simulink model "Finishonlyautomomous_v1"  (R2023b)
settings: Solver=FixedStepAuto  StartTime=0.0  StopTime=inf  RelTol=1e-3
libraries: vexarmcortexlib x6, vexcommonlib x2
settings Model: SimulationMode=external  ExtModeTrigDuration=25  Creator=nicoa  LastModifiedBy=ierdn
settings SolverCC: AlgebraicLoopSolver=TrustRegion
settings OptimizationCC: EnhancedBackFolding=on  PassReuseOutputArgsAs=Individual arguments  ZeroExternalMemoryAtStartup=off  ZeroInternalMemoryAtStartup=off  MaxStackSize=64  OptimizeBlockOrder=speed  DifferentSizesBufferReuse=on  OptimizationCustomize=off  EfficientTunableParamExpr=on
settings DebuggingCC: ParameterTunabilityLossMsg=error  UnconnectedInputMsg=warning  UnconnectedOutputMsg=warning  UnconnectedLineMsg=warning
settings HardwareCC: ProdBitPerPointer=32  ProdBitPerSizeT=32  ProdBitPerPtrDiffT=32  ProdLargestAtomicInteger=Long  ProdLargestAtomicFloat=Double  ProdWordSize=32  ProdHWDeviceType=ARM Compatible->ARM Cortex
settings ModelReferenceCC: EnableRefExpFcnMdlSchedulingChecks=on
settings SFSimCC: MATLABDynamicMemAlloc=off
settings RTWCC: Description=Embedded Coder  SystemTargetFile=ert.tlc  HardwareBoard=ARM Cortex-based VEX Microcontroller  TLCOptions="-aInlineSetEventsForThisBaseRateFcn=TLC_FALSE -aSuppressMultiTaskScheduler=TLC_FALSE  -aRateBasedStepFcn=0"  TemplateMakefile=ert_default_tmf  GenerateReport=on  Toolchain=GNU Tools for VEX ARM Cortex  IncludeHyperlinkInReport=on  LaunchReport=on  GenerateTraceInfo=on  GenerateTraceReport=on  GenerateTraceReportSl=on  GenerateTraceReportSf=on  GenerateTraceReportEml=on
settings CodeAppCC: ForceParamTrailComments=on  IgnoreCustomStorageClasses=off  OperatorAnnotations=on  SimulinkDataObjDesc=on  SFDataObjDesc=on  InsertBlockDesc=on
settings ERTTargetCC: ExtMode=on  ExtModeTransport=1  ExtModeMexFile=ext_serial_win32_comm  ExtModeMexArgs=1 3 115200

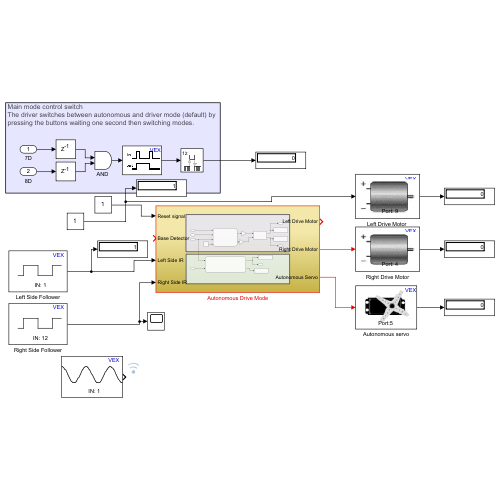
[thumbnail: Simulink's stored preview of the top-level diagram]
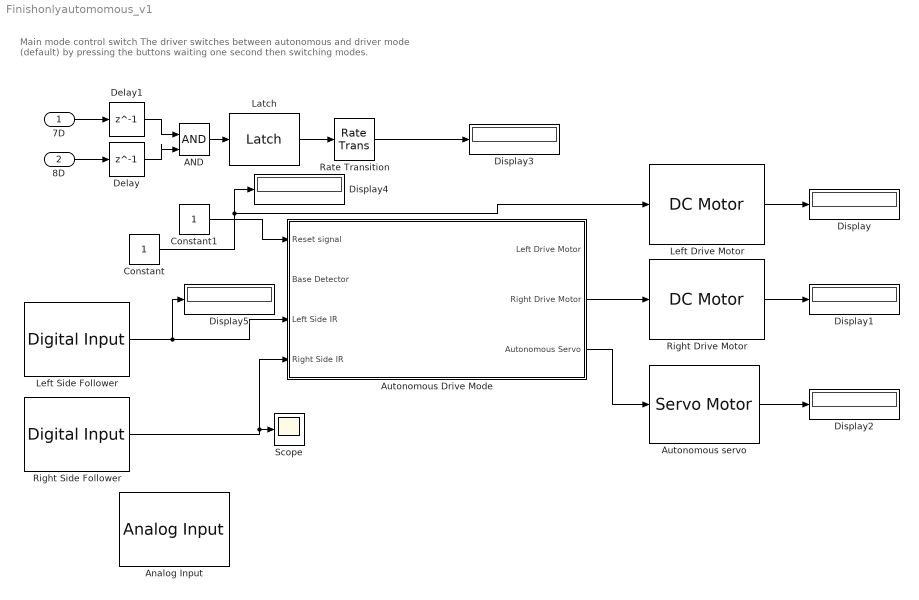
== system Finishonlyautomomous_v1 ==
  note: Main mode control switch
      | The driver switches between autonomous and driver mode (default) by
      | pressing the buttons waiting one second then switching modes.
  7D : Inport
  8D : Inport  Port=2
  "AND " : Logic  IconShape=distinctive  AllPortsSameDT=off  OutDataTypeStr=boolean
  Analog Input : vexarmcortexlib/Sensors/Analog Input  inChan=1  SimulationIn=off  SampleTime=0.05
  Autonomous Drive Mode : Subsystem
  Autonomous servo : vexarmcortexlib/Actuators/Servo Motor  motor=5  scaleFactor=60/127  SimulationOut=on
  Constant : Constant
  Constant1 : Constant
  Delay : Delay  DelayLength=1  InitialCondition=0  SampleTime=1
  Delay1 : Delay  DelayLength=1  InitialCondition=0  SampleTime=1
  Display{,1..5} (6 alike) : Display
  Latch : vexcommonlib/Latch  output0=off  BlockPlatform=vexarmcortex
  "Left Drive Motor " : vexarmcortexlib/Actuators/DC Motor  motor=9  scaleFactor=1/13.5  SimulationOut=on
  Left Side Follower : vexarmcortexlib/Sensors/Digital Input  inChan=1  SimulationIn=off  SampleTime=0.2
  Rate Transition : RateTransition
  Right Drive Motor : vexarmcortexlib/Actuators/DC Motor  motor=4  scaleFactor=1/13.5  SimulationOut=on
  Right Side Follower : vexarmcortexlib/Sensors/Digital Input  inChan=12  SimulationIn=off  SampleTime=0.2
  Scope : Scope
  wires:
  Delay1/1 -> "AND "/1
  "AND "/1 -> Latch/1
  7D/1 -> Delay1/1
  8D/1 -> Delay/1
  Latch/1 -> Rate Transition/1
  Delay/1 -> "AND "/2
  Right Side Follower/1 -> Scope/1, Autonomous Drive Mode/4(Right Side IR)
  Left Side Follower/1 -> Display5/1, Autonomous Drive Mode/3(Left Side IR)
  Constant/1 -> "Left Drive Motor "/1, Display4/1
  Autonomous Drive Mode/2(Right Drive Motor) -> Right Drive Motor/1
  Autonomous Drive Mode/3(Autonomous Servo) -> Autonomous servo/1
  "Left Drive Motor "/1 -> Display/1
  Right Drive Motor/1 -> Display1/1
  Autonomous servo/1 -> Display2/1
  Rate Transition/1 -> Display3/1
  Constant1/1 -> Autonomous Drive Mode/1(Reset signal)

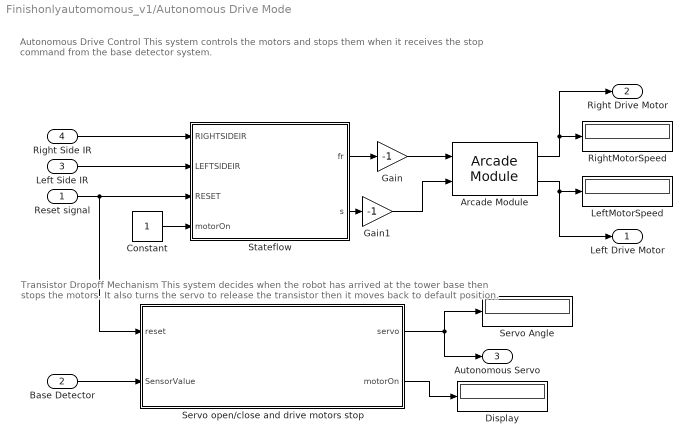
== system Finishonlyautomomous_v1/Autonomous Drive Mode ==
  note: Transistor Dropoff Mechanism
      | This system decides when the robot has arrived at the tower base then stops the motors. It also turns the servo to
      | release the transistor then it moves back to default position.
  note: Autonomous Drive Control
      | This system controls the motors and stops them when it receives the stop command from the base detector system.
  Reset signal : Inport
  Base Detector : Inport  Port=2
  Left Side IR : Inport  Port=3
  Right Side IR : Inport  Port=4
  Arcade Module : vexcommonlib/Arcade Module  BlockPlatform=vexarmcortex
  Constant : Constant
  Display : Display
  Gain : Gain  Gain=-1
  Gain1 : Gain  Gain=-1
  LeftMotorSpeed : Display
  RightMotorSpeed : Display
  Servo Angle : Display
  Servo open/close and drive motors stop : Stateflow chart  TreatAsAtomicUnit=on
  Stateflow : Stateflow chart  TreatAsAtomicUnit=on
  Left Drive Motor : Outport
  Right Drive Motor : Outport  Port=2
  Autonomous Servo : Outport  Port=3
  wires:
  Base Detector/1 -> Servo open/close and drive motors stop/2(SensorValue)
  Left Side IR/1 -> Stateflow/2(LEFTSIDEIR)
  Stateflow/1(fr) -> Gain/1
  Arcade Module/1 -> RightMotorSpeed/1, Right Drive Motor/1
  Arcade Module/2 -> LeftMotorSpeed/1, Left Drive Motor/1
  Servo open/close and drive motors stop/1(servo) -> Autonomous Servo/1, Servo Angle/1
  Reset signal/1 -> Servo open/close and drive motors stop/1(reset), Stateflow/3(RESET)
  Right Side IR/1 -> Stateflow/1(RIGHTSIDEIR)
  Constant/1 -> Stateflow/4(motorOn)
  Servo open/close and drive motors stop/2(motorOn) -> Display/1
  Gain/1 -> Arcade Module/1
  Stateflow/2(s) -> Gain1/1
  Gain1/1 -> Arcade Module/2

== stateflow chart Finishonlyautomomous_v1/Autonomous Drive Mode/Stateflow ==
  state STRAIGHT
    entry:
    fr = 40;
    s = 0;
  state GO_RIGHT
    entry:
    fr = 20
    s = 20;
  state GO_LEFT
    entry:
    fr = 20;
    s = -20;
  state STOP
    entry:
    fr = 0;
    s = 0;
  (default) -> STRAIGHT
  GO_LEFT -> STRAIGHT [order 3] : [LEFTSIDEIR == 1 && RIGHTSIDEIR == 1]
  GO_RIGHT -> STRAIGHT [order 3] : [RIGHTSIDEIR == 1 && LEFTSIDEIR == 1]
  STRAIGHT -> GO_RIGHT [order 3] : [RIGHTSIDEIR == 1 && LEFTSIDEIR == 0]
  STRAIGHT -> GO_LEFT [order 2] : [LEFTSIDEIR == 1 && RIGHTSIDEIR ==0]
  STOP -> STRAIGHT [order 3] : [RIGHTSIDEIR == 1 && LEFTSIDEIR == 1 && RESET == 0]
  STRAIGHT -> STOP [order 1] : [motorOn == 0]
  GO_LEFT -> GO_RIGHT [order 2] : [LEFTSIDEIR == 1 && RIGHTSIDEIR ==0]
  GO_RIGHT -> GO_LEFT [order 2] : [RIGHTSIDEIR == 1 && LEFTSIDEIR ==0]
  STOP -> GO_LEFT [order 2] : [RESET == 0 && LEFTSIDEIR == 1]
  GO_LEFT -> STOP [order 1] : [motorOn == 0]
  GO_RIGHT -> STOP [order 1] : [motorOn == 0]
  STOP -> GO_RIGHT [order 1] : [RESET == 0 && RIGHTSIDEIR == 1]
  data: RIGHTSIDEIR input; LEFTSIDEIR input; RESET input; motorOn input; fr output; s output

== stateflow chart Finishonlyautomomous_v1/Autonomous Drive Mode/Servo open//close and drive motors stop ==
  state move
    entry:
    servo = 0;
    motorOn = 1;
  state Stop
    entry:
    servo = 67;
    motorOn = 0;
  state off
    entry:
    servo = 0;
    motorOn = 0;
  (default) -> move
  off -> move : [reset == 0]
  move -> Stop : [SensorValue == 1]
  Stop -> off : [after(3,sec)]
  data: reset input; SensorValue input; servo output; motorOn output
